simulink model "Single_Core"  (R2025a)
settings: Solver=FixedStepDiscrete  StartTime=0.0  StopTime=20  RelTol=1e-3
libraries: simulink x1
settings Model: Creator=Ananthan  LastModifiedBy=Ananthan
settings DebuggingCC: AlgebraicLoopMsg=error

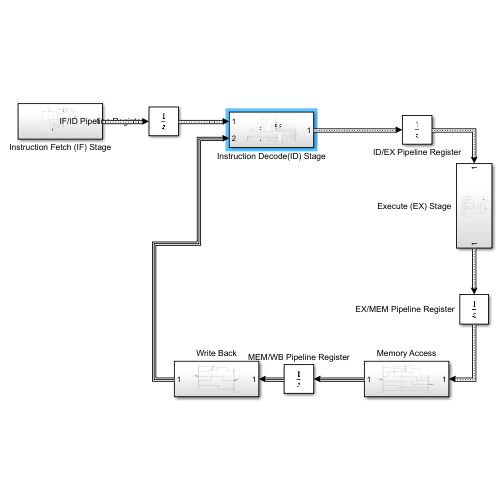
[thumbnail: Simulink's stored preview of the top-level diagram]
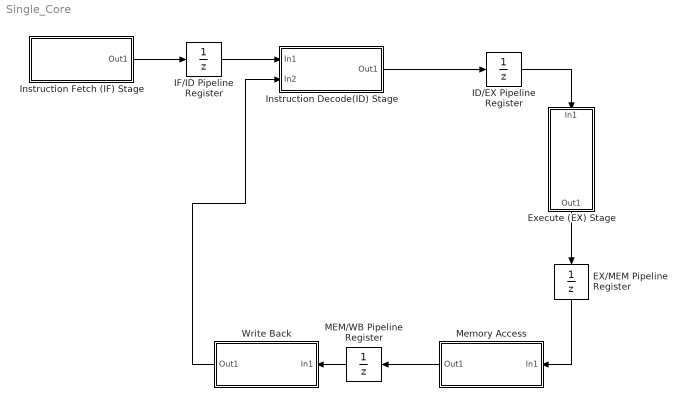
== system Single_Core ==
  EX/MEM Pipeline Register : UnitDelay  HasFrameUpgradeWarning=on
  Execute (EX) Stage : Subsystem
  ID/EX Pipeline Register : UnitDelay  HasFrameUpgradeWarning=on
  IF/ID Pipeline Register : UnitDelay  HasFrameUpgradeWarning=on
  Instruction Decode(ID) Stage : Subsystem
  Instruction Fetch (IF) Stage : Subsystem
  MEM/WB Pipeline Register : UnitDelay  HasFrameUpgradeWarning=on
  Memory Access : Subsystem
  Write Back : Subsystem
  wires:
  ID/EX Pipeline Register/1 -> Execute (EX) Stage/1(In1)
  Execute (EX) Stage/1(Out1) -> EX/MEM Pipeline Register/1
  EX/MEM Pipeline Register/1 -> Memory Access/1(In1)
  Memory Access/1(Out1) -> MEM/WB Pipeline Register/1
  Write Back/1(Out1) -> Instruction Decode(ID) Stage/2(In2)
  Instruction Fetch (IF) Stage/1(Out1) -> IF/ID Pipeline Register/1
  IF/ID Pipeline Register/1 -> Instruction Decode(ID) Stage/1(In1)
  MEM/WB Pipeline Register/1 -> Write Back/1(In1)
  Instruction Decode(ID) Stage/1(Out1) -> ID/EX Pipeline Register/1

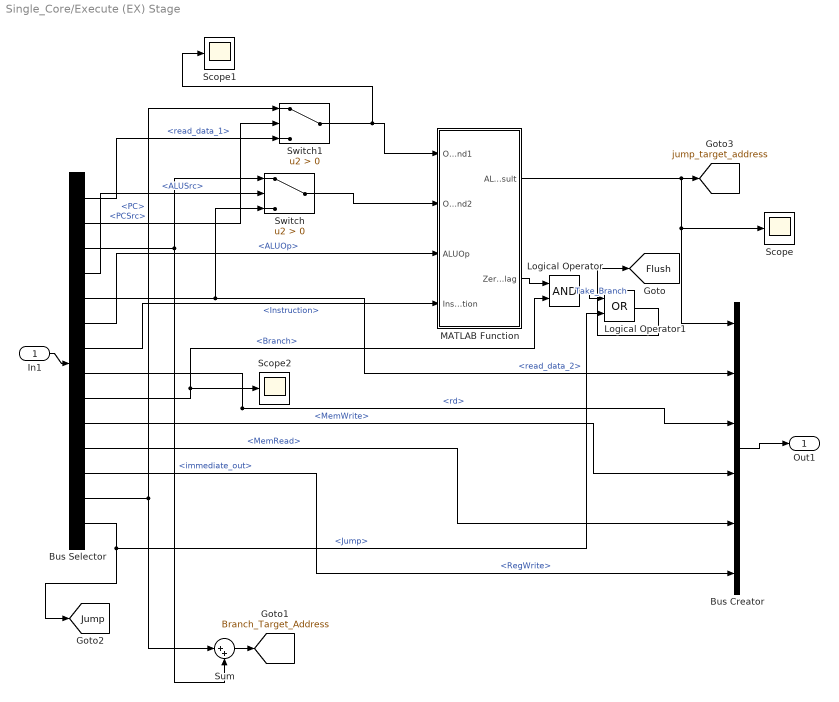
== system Single_Core/Execute (EX) Stage ==
  In1 : Inport
  Bus Creator : BusCreator  Inputs=6  OutDataTypeStr=Bus: EXMEM_Bus  NonVirtualBus=on
  Bus Selector : BusSelector  OutputSignals=read_data_1,PCSrc,immediate_out,ALUSrc,read_data_2,ALUOp,Instruction,rd,Branch,MemWrite,MemRead,RegWrite,PC,Jump
  Logical Operator : Logic  AllPortsSameDT=off  OutDataTypeStr=boolean
  Logical Operator1 : Logic  Operator=OR  AllPortsSameDT=off  OutDataTypeStr=boolean
  MATLAB Function : MATLAB Function  TreatAsAtomicUnit=on
  Scope : Scope
      settings: ActiveDisplayYMinimum=-14.39801238948076  ActiveDisplayYMaximum=30.01722157267616
  Scope1 : Scope
      settings: ActiveDisplayYMinimum=91.787947621079041  ActiveDisplayYMaximum=102.5794088339111
  Scope2 : Scope
      settings: ActiveDisplayYMinimum=-10.291310820308553  ActiveDisplayYMaximum=8.1075767531802825  DataLoggingVariableName=ScopeData2
  Sum : Sum  Inputs=|++
  Switch : Switch  Criteria=u2 > Threshold  OutDataTypeStr=int32  SaturateOnIntegerOverflow=off  InputSameDT=off
  Switch1 : Switch  Criteria=u2 > Threshold  OutDataTypeStr=int32  SaturateOnIntegerOverflow=off  InputSameDT=off
  Out1 : Outport
  tag scope: Branch_Target_Address=global, Flush=global, Jump=global, jump_target_address=global
  wires:
  Bus Creator/1 -> Out1/1
  In1/1 -> Bus Selector/1
  Bus Selector/3 -> Switch/1, Sum/2  "<immediate_out>"
  Bus Selector/8 -> Bus Creator/3  "<rd>"
  Bus Selector/5 -> Switch/3, Bus Creator/2  "<read_data_2>"
  Bus Selector/1 -> Switch1/3  "<read_data_1>"
  Bus Selector/6 -> MATLAB Function/3(ALUOp)  "<ALUOp>"
  Bus Selector/14 -> [Jump], Logical Operator1/2  "<Jump>"
  Bus Selector/9 -> Logical Operator/2, Scope2/1  "<Branch>"
  Bus Selector/10 -> Bus Creator/4  "<MemWrite>"
  Bus Selector/11 -> Bus Creator/5  "<MemRead>"
  Bus Selector/4 -> Switch/2  "<ALUSrc>"
  Bus Selector/12 -> Bus Creator/6  "<RegWrite>"
  Bus Selector/7 -> MATLAB Function/4(Instruction)  "<Instruction>"
  Switch/1 -> MATLAB Function/2(Operand2)
  MATLAB Function/1(ALU_Result) -> Scope/1, Bus Creator/1, [jump_target_address]
  MATLAB Function/2(Zero_Flag) -> Logical Operator/1
  Logical Operator/1 -> Logical Operator1/1  "Take_Branch"
  Bus Selector/13 -> Sum/1, Switch1/1  "<PC>"
  Sum/1 -> [Branch_Target_Address]
  Bus Selector/2 -> Switch1/2  "<PCSrc>"
  Switch1/1 -> Scope1/1, MATLAB Function/1(Operand1)
  Logical Operator1/1 -> [Flush]

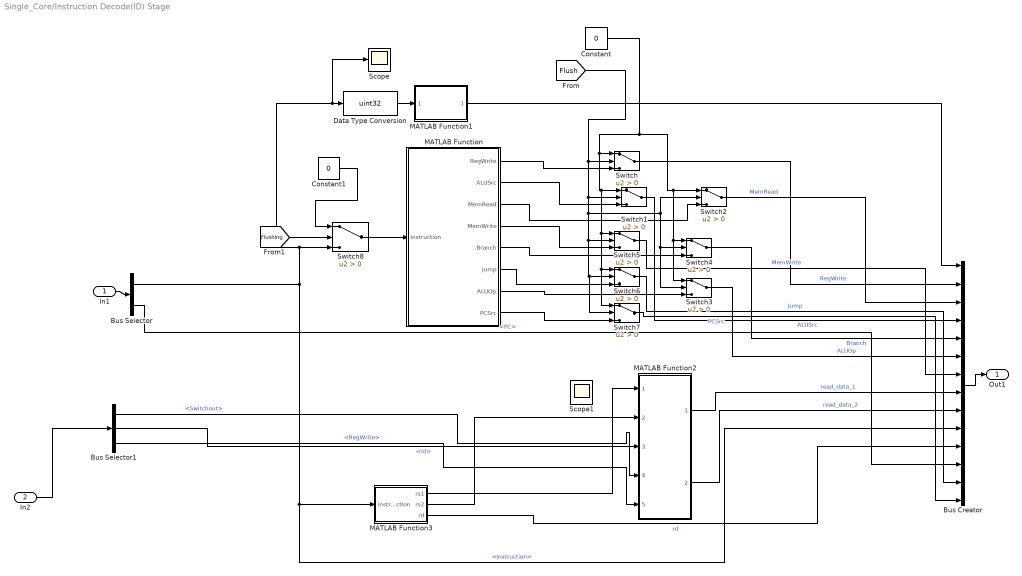
== system Single_Core/Instruction Decode(ID) Stage ==
  In1 : Inport
  In2 : Inport  Port=2
  Bus Creator : BusCreator  Inputs=14  OutDataTypeStr=Bus: IDEX_Bus  NonVirtualBus=on
  Bus Selector : BusSelector  OutputSignals=Instruction,PC
  Bus Selector1 : BusSelector  OutputSignals=Switchout,rd,RegWrite
  Constant : Constant  Value=0  OutDataTypeStr=uint8
  Constant1 : Constant  Value=0
  Data Type Conversion : DataTypeConversion  OutDataTypeStr=uint32  SaturateOnIntegerOverflow=off  RndMeth=Floor
  MATLAB Function : MATLAB Function  TreatAsAtomicUnit=on
  MATLAB Function1 : MATLAB Function  TreatAsAtomicUnit=on
  MATLAB Function2 : MATLAB Function  TreatAsAtomicUnit=on
  MATLAB Function3 : MATLAB Function  TreatAsAtomicUnit=on
  Scope : Scope
      settings: ActiveDisplayYMinimum=-9.62360957507877E+7  ActiveDisplayYMaximum=2.9515143357319188E+8  DataLoggingVariableName=ScopeData4
  Scope1 : Scope
      settings: ActiveDisplayYMinimum=-1.0224235765954815E+6  ActiveDisplayYMaximum=2.6269684460485624E+6  DataLoggingVariableName=ScopeData5
  Switch{,1..5,7} (7 alike) : Switch  Criteria=u2 > Threshold  OutDataTypeStr=uint32  SaturateOnIntegerOverflow=off  InputSameDT=off
  Switch6 : Switch  Criteria=u2 > Threshold  OutDataTypeStr=boolean  SaturateOnIntegerOverflow=off  InputSameDT=off
  Switch8 : Switch  Criteria=u2 > Threshold  SaturateOnIntegerOverflow=off  InputSameDT=off
  Out1 : Outport
  wires:
  Bus Creator/1 -> Out1/1
  In1/1 -> Bus Selector/1
  Bus Selector/1 -> Scope/1, Data Type Conversion/1, Switch8/3, MATLAB Function3/1(instruction), Bus Creator/10  "<Instruction>"
  MATLAB Function2/1(ReadData1) -> Bus Creator/8  "read_data_1"
  MATLAB Function2/2(ReadData2) -> Bus Creator/9  "read_data_2"
  MATLAB Function1/1(immediate_out) -> Bus Creator/1
  MATLAB Function3/3(rd) -> Bus Creator/11  "rd"
  MATLAB Function/7(ALUOp) -> Switch3/3
  MATLAB Function/6(Jump) -> Switch6/3
  MATLAB Function/5(Branch) -> Switch4/3
  MATLAB Function/4(MemWrite) -> Switch5/3
  MATLAB Function/3(MemRead) -> Switch2/3
  MATLAB Function/2(ALUSrc) -> Switch1/3
  Bus Selector1/2 -> MATLAB Function2/3(WriteAddr)  "<rd>"
  Bus Selector1/3 -> MATLAB Function2/5(WriteEnable)  "<RegWrite>"
  Bus Selector1/1 -> MATLAB Function2/4(WriteData)  "<Switchout>"
  MATLAB Function3/2(rs2) -> MATLAB Function2/2(ReadAddr2)
  Bus Selector/2 -> Bus Creator/12  "<PC>"
  MATLAB Function/8(PCSrc) -> Switch7/3
  MATLAB Function/1(RegWrite) -> Switch/3
  [Flush] -> Switch1/2, Switch3/2, Switch4/2, Switch2/2, Switch7/2, Switch6/2, Switch5/2, Switch/2
  Constant/1 -> Switch3/1, Switch4/1, Switch2/1, Switch7/1, Switch6/1, Switch5/1, Switch1/1, Switch/1
  Switch/1 -> Bus Creator/2  "RegWrite"
  Switch2/1 -> Bus Creator/3  "MemRead"
  Switch1/1 -> Bus Creator/4  "ALUSrc"
  Switch4/1 -> Bus Creator/5  "Branch"
  Switch3/1 -> Bus Creator/6  "ALUOp"
  Switch5/1 -> Bus Creator/7  "MemWrite"
  Switch6/1 -> Bus Creator/13  "Jump"
  Switch7/1 -> Bus Creator/14  "PCSrc"
  MATLAB Function3/1(rs1) -> MATLAB Function2/1(ReadAddr1)
  In2/1 -> Bus Selector1/1
  Switch8/1 -> MATLAB Function/1(instruction)
  Constant1/1 -> Switch8/1
  [Flushing] -> Switch8/2
  Data Type Conversion/1 -> MATLAB Function1/1(instruction)

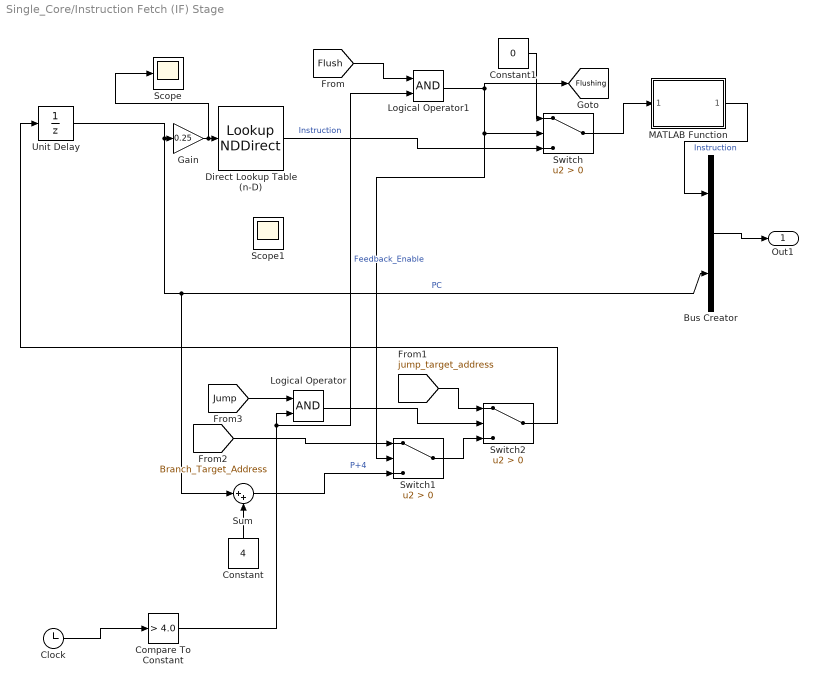
== system Single_Core/Instruction Fetch (IF) Stage ==
  Bus Creator : BusCreator  Inputs=2  OutDataTypeStr=Bus: IFID_Bus  NonVirtualBus=on
  Clock : Clock
  Compare To Constant : simulink/Logic and Bit Operations/Compare To Constant  relop=>  const=4.0  OutDataTypeStr=boolean
  Constant : Constant  Value=4
  Constant1 : Constant  Value=0
  Direct Lookup Table (n-D) : LookupNDDirect  NumberOfTableDimensions=1  Table=[12583059;1056803;8451;4293984531;2105379;1122707;4261513443;32871;0;0]  DiagnosticForOutOfRangeInput=Error  TableDataTypeStr=fixdt('uint32', 'DataTypeOverride', 'Off')
  Gain : Gain  Gain=0.25  OutDataTypeStr=uint8
  Logical Operator : Logic  AllPortsSameDT=off  OutDataTypeStr=boolean
  Logical Operator1 : Logic  AllPortsSameDT=off  OutDataTypeStr=boolean
  MATLAB Function : MATLAB Function  TreatAsAtomicUnit=on
  Scope : Scope
      settings: ActiveDisplayYMinimum=-3.5050370179398769  ActiveDisplayYMaximum=12.885568928882551  DataLoggingVariableName=ScopeData3
  Scope1 : Scope
      settings: ActiveDisplayYMinimum=17.53381287399019  ActiveDisplayYMaximum=50.599648083752676  DataLoggingVariableName=ScopeData6
  Sum : Sum  Inputs=|++  OutDataTypeStr=uint32  AccumDataTypeStr=uint32
  Switch : Switch  Criteria=u2 > Threshold  OutDataTypeStr=uint32  SaturateOnIntegerOverflow=off  InputSameDT=off
  Switch1 : Switch  Criteria=u2 > Threshold  OutDataTypeStr=uint8  SaturateOnIntegerOverflow=off  InputSameDT=off
  Switch2 : Switch  Criteria=u2 > Threshold  OutDataTypeStr=uint32  SaturateOnIntegerOverflow=off  InputSameDT=off
  Unit Delay : UnitDelay  HasFrameUpgradeWarning=on
  Out1 : Outport
  tag scope: Flushing=global
  wires:
  Unit Delay/1 -> Gain/1, Bus Creator/2, Sum/1  "PC"
  Constant/1 -> Sum/2
  Direct Lookup Table (n-D)/1 -> Switch/3  "Instruction"
  [jump_target_address] -> Switch2/1
  Logical Operator1/1 -> Switch/2, Switch1/2, [Flushing]
  Sum/1 -> Switch1/3  "P+4"
  Bus Creator/1 -> Out1/1
  Switch1/1 -> Switch2/3
  Switch2/1 -> Unit Delay/1
  [Jump] -> Logical Operator/1
  [Branch_Target_Address] -> Switch1/1
  Clock/1 -> Compare To Constant/1
  Compare To Constant/1 -> Logical Operator1/2, Logical Operator/2  "Feedback_Enable"
  Logical Operator/1 -> Switch2/2
  [Flush] -> Logical Operator1/1
  Gain/1 -> Scope/1, Direct Lookup Table (n-D)/1
  MATLAB Function/1(scalar_out) -> Bus Creator/1  "Instruction"
  Switch/1 -> MATLAB Function/1(vector_in)
  Constant1/1 -> Switch/1

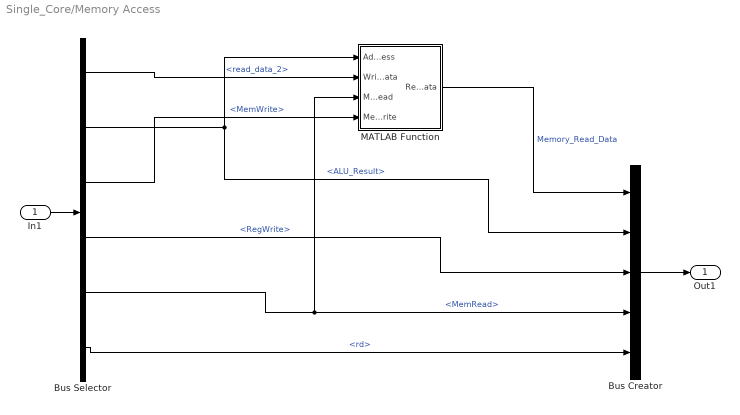
== system Single_Core/Memory Access ==
  In1 : Inport
  Bus Creator : BusCreator  Inputs=5  OutDataTypeStr=Bus: MEMWB_Bus
  Bus Selector : BusSelector  OutputSignals=read_data_2,ALU_Result,MemWrite,RegWrite,MemRead,rd
  MATLAB Function : MATLAB Function  TreatAsAtomicUnit=on
  Out1 : Outport
  wires:
  In1/1 -> Bus Selector/1
  Bus Selector/2 -> MATLAB Function/1(Address), Bus Creator/2  "<ALU_Result>"
  Bus Selector/6 -> Bus Creator/5  "<rd>"
  Bus Selector/3 -> MATLAB Function/4(MemWrite)  "<MemWrite>"
  Bus Selector/5 -> MATLAB Function/3(MemRead), Bus Creator/4  "<MemRead>"
  Bus Selector/4 -> Bus Creator/3  "<RegWrite>"
  Bus Selector/1 -> MATLAB Function/2(WriteData)  "<read_data_2>"
  MATLAB Function/1(ReadData) -> Bus Creator/1  "Memory_Read_Data"
  Bus Creator/1 -> Out1/1

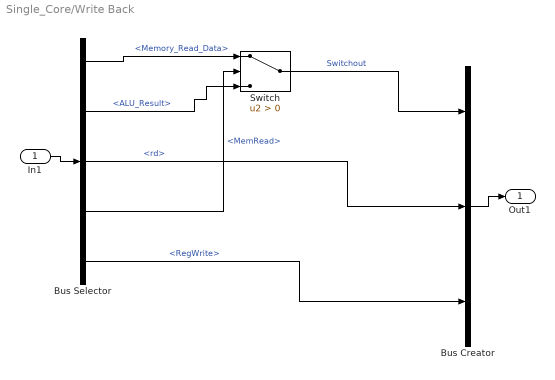
== system Single_Core/Write Back ==
  In1 : Inport
  Bus Creator : BusCreator  Inputs=3
  Bus Selector : BusSelector  OutputSignals=Memory_Read_Data,ALU_Result,rd,MemRead,RegWrite
  Switch : Switch  Criteria=u2 > Threshold  SaturateOnIntegerOverflow=off  InputSameDT=off
  Out1 : Outport
  wires:
  Bus Creator/1 -> Out1/1
  In1/1 -> Bus Selector/1
  Bus Selector/1 -> Switch/1  "<Memory_Read_Data>"
  Bus Selector/3 -> Bus Creator/2  "<rd>"
  Bus Selector/4 -> Switch/2  "<MemRead>"
  Bus Selector/5 -> Bus Creator/3  "<RegWrite>"
  Bus Selector/2 -> Switch/3  "<ALU_Result>"
  Switch/1 -> Bus Creator/1  "Switchout"

== matlab function Single_Core/Instruction Decode(ID) Stage/MATLAB Function1 ==
  data: instruction input uint32; immediate_out output int32
function immediate_out = immediate_generator(instruction)
% This function generates a 32-bit sign-extended immediate.
% It uses a robust subtraction method for sign extension to prevent
% type conversion errors in the Simulink Coder.

    instr = uint32(instruction);
    opcode = bitand(instr, uint32(127));

    % Define opcodes
    OPCODE_I_TYPE   = uint32(hex2dec('13'));
    OPCODE_LOAD     = uint32(hex2dec('03'));
    OPCODE_JALR     = uint32(hex2dec('67'));
    OPCODE_STORE    = uint32(hex2dec('23'));
    OPCODE_BRANCH   = uint32(hex2dec('63'));
    OPCODE_LUI      = uint32(hex2dec('37'));
    OPCODE_JAL      = uint32(hex2dec('6F'));

    imm_val = int32(0); % Use a signed integer for the final value
    
    switch opcode
        case {OPCODE_I_TYPE, OPCODE_LOAD, OPCODE_JALR} % I-type
            imm_unsigned = bitshift(instr, -20);
            sign_bit = bitget(imm_unsigned, 12);
            if sign_bit
                % Two's complement: val - 2^12
                imm_val = int32(imm_unsigned) - 4096; 
            else
                imm_val = int32(imm_unsigned);
            end

        case OPCODE_STORE % S-type
            imm_11_5 = bitshift(instr, -25);
            imm_4_0  = bitshift(bitand(instr, uint32(hex2dec('F80'))), -7);
            imm_unsigned = bitor(imm_11_5, imm_4_0);
            sign_bit = bitget(imm_unsigned, 12);
            if sign_bit
                imm_val = int32(imm_unsigned) - 4096;
            else
                imm_val = int32(imm_unsigned);
            end
            
        case OPCODE_BRANCH % B-type
            imm_12   = bitshift(bitand(instr, uint32(hex2dec('80000000'))), -19);
            imm_10_5 = bitshift(bitand(instr, uint32(hex2dec('7E000000'))), -20);
            imm_4_1  = bitshift(bitand(instr, uint32(hex2dec('F00'))), -7);
            imm_11   = bitshift(bitand(instr, uint32(hex2dec('80'))), 4);
            imm_unsigned = bitor(bitor(bitor(imm_12, imm_11), imm_10_5), imm_4_1);
            sign_bit = bitget(imm_unsigned, 13);
            if sign_bit
                imm_val = int32(imm_unsigned) - 8192; % 2^13
            else
                imm_val = int32(imm_unsigned);
            end
        
        case OPCODE_LUI % U-type
            imm_val = int32(bitand(instr, uint32(hex2dec('FFFFF000'))));

        case OPCODE_JAL % J-type
            imm_20   = bitshift(bitand(instr, uint32(hex2dec('80000000'))), -11);
            imm_10_1 = bitshift(bitand(instr, uint32(hex2dec('7FE00000'))), -20);
            imm_11   = bitshift(bitand(instr, uint32(hex2dec('100000'))), -9);
            imm_19_12= bitand(instr, uint32(hex2dec('FF000')));
            imm_unsigned = bitor(bitor(bitor(imm_20, imm_19_12), imm_11), imm_10_1);
            sign_bit = bitget(imm_unsigned, 21);
            if sign_bit
                imm_val = int32(imm_unsigned) - 2097152; % 2^21
            else
                imm_val = int32(imm_unsigned);
            end
    end
    
    immediate_out = imm_val;
end

== matlab function Single_Core/Instruction Decode(ID) Stage/MATLAB Function ==
  data: instruction input; RegWrite output; ALUSrc output; MemRead output; MemWrite output; Branch output; Jump output boolean; ALUOp output; PCSrc output
function [RegWrite, ALUSrc, MemRead, MemWrite, Branch, Jump, ALUOp, PCSrc] = control_unit(instruction)
% This is the final, complete, and fully corrected Control Unit code.

    instr = uint32(instruction);
    
    % Define opcodes for different instruction types
    OPCODE_R_TYPE   = uint32(hex2dec('33')); % R-type (add, sub, etc.)
    OPCODE_I_TYPE   = uint32(hex2dec('13')); % I-type (addi, etc.)
    OPCODE_LOAD     = uint32(hex2dec('03')); % Load (lw)
    OPCODE_STORE    = uint32(hex2dec('23')); % Store (sw)
    OPCODE_BRANCH   = uint32(hex2dec('63')); % Branch (beq)
    OPCODE_JAL      = uint32(hex2dec('6F')); % Jump and Link
    OPCODE_JALR     = uint32(hex2dec('67')); % Jump and Link Register
    OPCODE_LUI      = uint32(hex2dec('37')); % Load Upper Immediate

    % Initialize all control signals to a default (inactive) state
    RegWrite = false;
    ALUSrc   = false; % Selects ALU Operand 2 (false=Register, true=Immediate)
    MemRead  = false;
    MemWrite = false;
    Branch   = false;
    Jump     = false;
    PCSrc    = false; % Selects ALU Operand 1 (false=Register, true=PC)
    ALUOp    = [0 0]; % ALU Operation category
    
    opcode = bitand(instr, uint32(127)); % Extract opcode

    % Decode the instruction
    switch opcode
        case OPCODE_R_TYPE
            RegWrite = true;
            ALUSrc   = false;
            PCSrc    = false;
            ALUOp    = [1 0]; 
        case OPCODE_I_TYPE
            RegWrite = true;
            ALUSrc   = true;
            PCSrc    = false;
            ALUOp    = [1 1];
        case OPCODE_LOAD
            RegWrite = true;
            ALUSrc   = true;
            MemRead  = true;
            PCSrc    = false;
            ALUOp    = [0 0];
        case OPCODE_STORE
            ALUSrc   = true;
            MemWrite = true;
            PCSrc    = false;
            ALUOp    = [0 0];
        case OPCODE_BRANCH
            Branch   = true;
            ALUSrc   = false;
            PCSrc    = false;
            ALUOp    = [0 1];
        case OPCODE_JAL
            RegWrite = true;
            Jump     = true;
            ALUSrc   = true;
            PCSrc    = true;  % FIX: Use PC as the first ALU operand
            ALUOp    = [0 0]; % ALU performs addition
        case OPCODE_JALR
            RegWrite = true;
            Jump     = true;
            ALUSrc   = true;
            PCSrc    = false; % Use register value as the first ALU operand
            ALUOp    = [0 0];
        case OPCODE_LUI
            RegWrite = true;
            ALUSrc   = true;
            PCSrc    = true;  % First operand can be PC (or 0), second is immediate
            ALUOp    = [0 0];
    end
end

== matlab function Single_Core/Execute (EX) Stage/MATLAB Function ==
  data: Operand1 input; ALU_Result output int32 size=1; Operand2 input; ALUOp input; Instruction input; Zero_Flag output boolean size=1
function [ALU_Result, Zero_Flag] = alu(Operand1, Operand2, ALUOp, Instruction)
% This function models the RISC-V ALU and its control unit.
% The logic within this function is correct.

    % Ensure inputs are of a consistent integer type for bitwise operations
    op1 = int32(Operand1);
    op2 = int32(Operand2);
    instr = uint32(Instruction);
    
    % Convert 2-bit vector to a decimal number using basic math
    alu_op_val = ALUOp(1)*2 + ALUOp(2); 

    % Extract funct3 and funct7 from the instruction
    funct3 = bitshift(bitand(instr, uint32(hex2dec('7000'))), -12);
    funct7 = bitshift(bitand(instr, uint32(hex2dec('FE000000'))), -25);

    % Default result
    ALU_Result = int32(0);

    % Main ALU operation decoding
    switch alu_op_val
        case 0 % '00' -> For LW, SW, ADDI
            ALU_Result = op1 + op2;
        case 1 % '01' -> For Branches
            ALU_Result = op1 - op2;
        case 2 % '10' -> R-type instructions
            switch funct3
                case 0 % ADD or SUB
                    if funct7 == 32, ALU_Result = op1 - op2; else, ALU_Result = op1 + op2; end
                case 1 % SLL
                    ALU_Result = int32(bitshift(uint32(op1), op2));
                case 2 % SLT
                    if op1 < op2, ALU_Result = int32(1); else, ALU_Result = int32(0); end
                case 4 % XOR
                    ALU_Result = bitxor(op1, op2);
                case 6 % OR
                    ALU_Result = bitor(op1, op2);
                case 7 % AND
                    ALU_Result = bitand(op1, op2);
                otherwise
                    ALU_Result = int32(0);
            end
        case 3 % '11' -> I-type instructions
             switch funct3
                case 0 % ADDI
                    ALU_Result = op1 + op2;
                case 2 % SLTI
                     if op1 < op2, ALU_Result = int32(1); else, ALU_Result = int32(0); end
                case 4 % XORI
                    ALU_Result = bitxor(op1, op2);
                case 6 % ORI
                    ALU_Result = bitor(op1, op2);
                case 7 % ANDI
                    ALU_Result = bitand(op1, op2);
                otherwise
                    ALU_Result = int32(0);
             end
    end
    
    % Set the Zero_Flag output
    Zero_Flag = (ALU_Result == 0);
end

== matlab function Single_Core/Instruction Decode(ID) Stage/MATLAB Function2 ==
  data: ReadAddr1 input; ReadData1 output int32; ReadAddr2 input; WriteAddr input; WriteData input; WriteEnable input; ReadData2 output int32
function [ReadData1, ReadData2] = register_file(ReadAddr1, ReadAddr2, WriteAddr, WriteData, WriteEnable)
% Implements a 32-register file for a RISC-V processor.
% x0 is hardwired to zero. Uses 1-based MATLAB indexing.

    persistent Registers;
    if isempty(Registers)
        Registers = zeros(32, 1, 'int32');
    end

    % 1. Handle the Write-Back from the WB stage first (synchronous write)
    if WriteEnable
        if WriteAddr > 0 % Do not write to register x0
            % MATLAB arrays are 1-based, so we add 1 to the 0-based RISC-V address
            Registers(WriteAddr + 1) = WriteData;
        end
    end

    % 2. Perform the Reads for the ID stage (combinational read)
    if ReadAddr1 == 0
        ReadData1 = int32(0);
    else
        ReadData1 = Registers(ReadAddr1 + 1);
    end

    if ReadAddr2 == 0
        ReadData2 = int32(0);
    else
        ReadData2 = Registers(ReadAddr2 + 1);
    end
end

== matlab function Single_Core/Memory Access/MATLAB Function ==
  data: Address input int32; WriteData input; MemRead input; MemWrite input; ReadData output int32
function ReadData = data_memory(Address, WriteData, MemRead, MemWrite)
% This function models a synchronous data memory that only accesses
% memory when a read or write signal is active.

    persistent Memory;
    if isempty(Memory)
        Memory = zeros(16384, 1, 'int32');
    end

    % Default output is 0
    ReadData = int32(0);
    
    % Only perform a memory operation if requested
    if MemRead || MemWrite
        % Convert the byte address to a 1-based word index
        wordAddress = (Address / 4) + 1;

        % Perform the read operation if requested
        if MemRead
            ReadData = Memory(wordAddress);
        end

        % Perform the write operation if requested
        if MemWrite
            Memory(wordAddress) = WriteData;
        end
    end
end

== matlab function Single_Core/Instruction Fetch (IF) Stage/MATLAB Function ==
  data: vector_in input; scalar_out output uint32
function scalar_out = to_scalar(vector_in)
% This function extracts the first element from an input vector
% and ensures the output is a uint32 scalar.
    scalar_out = uint32(vector_in(1));
end

== matlab function Single_Core/Instruction Decode(ID) Stage/MATLAB Function3 ==
  data: instruction input; rs1 output uint8; rs2 output uint8; rd output uint8
function [rs1, rs2, rd] = bit_slicer(instruction)
% This function correctly extracts the rs1, rs2, and rd fields
% from a 32-bit RISC-V instruction word.

    instr = uint32(instruction);

    % Extract rd (destination register, bits 11:7)
    rd  = uint8(bitshift(bitand(instr, uint32(hex2dec('F80'))), -7));

    % Extract rs1 (source register 1, bits 19:15)
    rs1 = uint8(bitshift(bitand(instr, uint32(hex2dec('F8000'))), -15));

    % Extract rs2 (source register 2, bits 24:20)
    rs2 = uint8(bitshift(bitand(instr, uint32(hex2dec('1F00000'))), -20));
end
